simulink model "MirrorSubsystemnor"  (R2018a)
settings: Solver=VariableStepAuto  StartTime=0.0  StopTime=10.0  RelTol=1e-3
libraries: simulink x4
settings Model: Creator=Sushma  LastModifiedBy=training
settings DataIOCC: ReturnWorkspaceOutputs=on
settings SFSimCC: SimUseLocalCustomCode=on
settings RTWCC: RTWUseLocalCustomCode=on

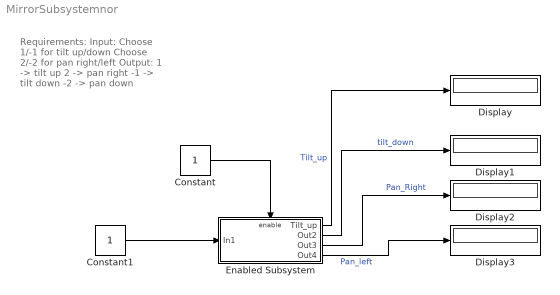
== system MirrorSubsystemnor ==
  note: Requirements:
      | Input:
      | Choose 1/-1 for tilt up/down
      | Choose 2/-2 for pan right/left
      | Output:
      | 1  ->  tilt up
      | 2  -> pan right
      | -1 -> tilt down
      | -2 -> pan down
  Constant : Constant
  Constant1 : Constant
  Display{,1..3} (4 alike) : Display
  Enabled Subsystem : Subsystem  TreatAsAtomicUnit=on
  wires:
  Enabled Subsystem/2(Out2) -> Display1/1  "tilt_down"
  Constant/1 -> Enabled Subsystem/Enable
  Enabled Subsystem/3(Out3) -> Display2/1  "Pan_Right"
  Enabled Subsystem/4(Out4) -> Display3/1  "Pan_left"
  Enabled Subsystem/1(Tilt_up) -> Display/1  "Tilt_up"
  Constant1/1 -> Enabled Subsystem/1(In1)

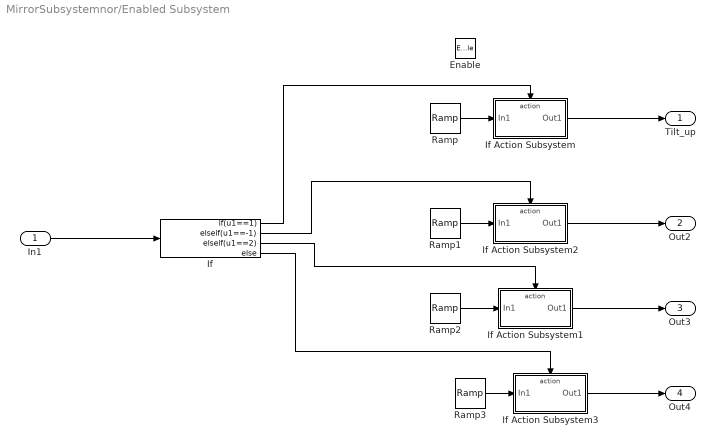
== system MirrorSubsystemnor/Enabled Subsystem ==
  In1 : Inport
  Enable : EnablePort
  If : If  IfExpression=u1==1  ElseIfExpressions=u1==-1 , u1==2
  If Action Subsystem : Subsystem  TreatAsAtomicUnit=on
  If Action Subsystem1 : Subsystem  TreatAsAtomicUnit=on
  If Action Subsystem2 : Subsystem  TreatAsAtomicUnit=on
  If Action Subsystem3 : Subsystem  TreatAsAtomicUnit=on
  Ramp : simulink/Sources/Ramp  slope=0  start=1  InitialOutput=0
  Ramp1 : simulink/Sources/Ramp  slope=0  start=-1  InitialOutput=0
  Ramp2 : simulink/Sources/Ramp  slope=0  start=0  InitialOutput=2
  Ramp3 : simulink/Sources/Ramp  slope=0  start=0  InitialOutput=-2
  Tilt_up : Outport
  Out2 : Outport  Port=2
  Out3 : Outport  Port=3
  Out4 : Outport  Port=4
  wires:
  If/1 -> If Action Subsystem/Action
  If/2 -> If Action Subsystem2/Action
  If/3 -> If Action Subsystem1/Action
  If/4 -> If Action Subsystem3/Action
  Ramp/1 -> If Action Subsystem/1(In1)
  If Action Subsystem/1(Out1) -> Tilt_up/1
  Ramp1/1 -> If Action Subsystem2/1(In1)
  Ramp2/1 -> If Action Subsystem1/1(In1)
  Ramp3/1 -> If Action Subsystem3/1(In1)
  If Action Subsystem2/1(Out1) -> Out2/1
  If Action Subsystem1/1(Out1) -> Out3/1
  If Action Subsystem3/1(Out1) -> Out4/1
  In1/1 -> If/1

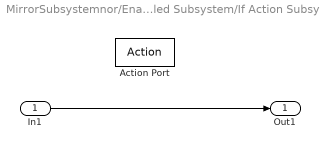
== system MirrorSubsystemnor/Enabled Subsystem/If Action Subsystem ==
  In1 : Inport
  Action Port : ActionPort
  Out1 : Outport
  wires:
  In1/1 -> Out1/1

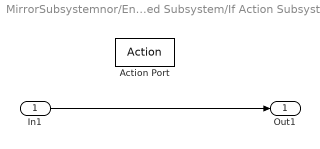
== system MirrorSubsystemnor/Enabled Subsystem/If Action Subsystem1 ==
  In1 : Inport
  Action Port : ActionPort
  Out1 : Outport
  wires:
  In1/1 -> Out1/1

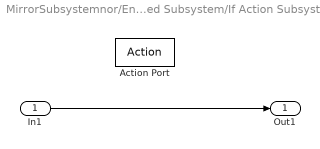
== system MirrorSubsystemnor/Enabled Subsystem/If Action Subsystem2 ==
  In1 : Inport
  Action Port : ActionPort
  Out1 : Outport
  wires:
  In1/1 -> Out1/1

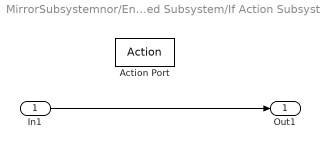
== system MirrorSubsystemnor/Enabled Subsystem/If Action Subsystem3 ==
  In1 : Inport
  Action Port : ActionPort
  Out1 : Outport
  wires:
  In1/1 -> Out1/1
